simulink model "RandomSpeed"  (Simulink 7.4)
settings: Solver=ode45  StartTime=0.0  StopTime=480  RelTol=1e-3
values from neighbouring files (symbols this model uses):
  speed = speed1(:,i)    [VGait_Input_Signals.m]
libraries: dsparch4 x1, commnoisgen2 x1
settings Model: Creator=Sandy  LastModifiedBy=Sandy

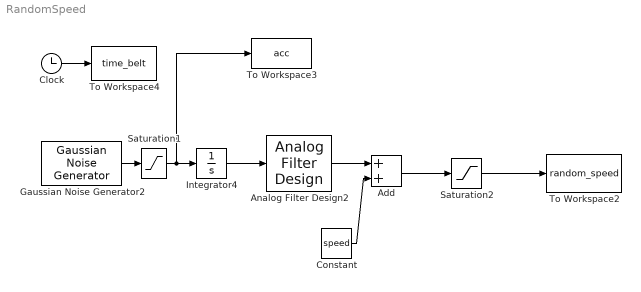
== system RandomSpeed ==
  Add : Sum  OutDataType=fixdt(1, 16)  OutScaling=2^-10
  Analog Filter Design2 : dsparch4/Analog Filter Design  method=Butterworth  filttype=Highpass  N=2  Wlo=fc  Whi=80  Rp=2  Rs=40
  Clock : Clock
      settings: Decimation=10
  Constant : Constant  Value=speed  OutDataType=fixdt(1, 16)  OutScaling=2^0
  Gaussian Noise Generator2 : commnoisgen2/Gaussian Noise Generator  SystemSampleTime=-1  m=0  d=var  s=41  Ts=0.0033  frameBased=off  sampPerFrame=1  orient=off  outDataType=double
  Integrator4 : Integrator
  Saturation1 : Saturate  UpperLimit=15  LowerLimit=-15  SampleTime=0.0033  OutDataType=fixdt(1, 16)  OutScaling=2^0
  Saturation2 : Saturate  UpperLimit=3.6  LowerLimit=0  SampleTime=0.0033  OutDataType=fixdt(1, 16)  OutScaling=2^0
  To Workspace2 : ToWorkspace  VariableName=random_speed  SampleTime=0.0033  SaveFormat=Array
  To Workspace3 : ToWorkspace  VariableName=acc  SampleTime=0.0033  SaveFormat=Array
  To Workspace4 : ToWorkspace  VariableName=time_belt  SampleTime=0.0033  SaveFormat=Array
  wires:
  Saturation2/1 -> To Workspace2/1
  Constant/1 -> Add/2
  Clock/1 -> To Workspace4/1
  Add/1 -> Saturation2/1
  Analog Filter Design2/1 -> Add/1
  Gaussian Noise Generator2/1 -> Saturation1/1
  Integrator4/1 -> Analog Filter Design2/1
  Saturation1/1 -> Integrator4/1, To Workspace3/1
